simulink model "A5_3_sampling_100ms"  (Simulink 7.4)
settings: Solver=FixedStepDiscrete  StartTime=0.0  StopTime=5  RelTol=1e-3
undefined symbols (not defined in the file): den, num
libraries: DCmotor_library x1
settings Model: Creator=Natalia  LastModifiedBy=ma
settings DebuggingCC: FcnCallInpInsideContextMsg=Enable All  StrictBusMsg=ErrorLevel1
settings HardwareCC: ProdIntDivRoundTo=Zero  ProdEndianess=LittleEndian  ProdHWDeviceType=Generic->32-bit x86 compatible
settings RTWCC: SystemTargetFile=rtwin.tlc  TemplateMakefile=rtwin.tmf  Description=Real-Time Windows Target  ProcessScript=rtwin_make_rtw_hook  RTWCompilerOptimization=On
settings CodeAppCC: MaxIdLength=95  CustomSymbolStrType=$N$R$M_T
settings TargetCC: TargetLibSuffix=_rtwin.lib  TargetPreCompLibLocation=C:\Program Files\MATLAB\R2012a\toolbox\rtw\targets\rtwin\lib\win64  TargetFunctionLibrary=ANSI_C  IsPILTarget=off  MatFileLogging=on  EnableShiftOperators=on
settings CustomProperty: DataType=string  Value=C:/PROGRA~1/MATLAB/R2012a/toolbox/rtw/targets/rtwin

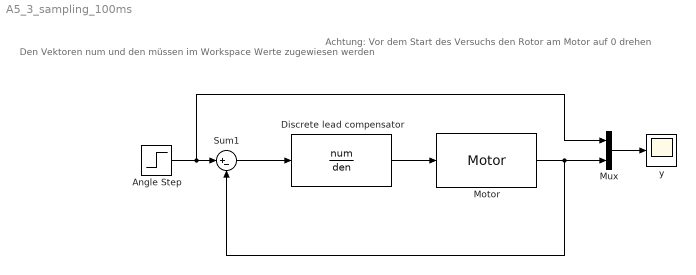
== system A5_3_sampling_100ms ==
  note: Den Vektoren
      | num und den
      | müssen im Workspace
      | Werte zugewiesen werden
  note: Achtung:
      | Vor dem Start des Versuchs
      | den Rotor am Motor auf 0 drehen
  Angle Step : Step  After=2*pi  SampleTime=0.1
  Discrete lead compensator : DiscreteTransferFcn  Numerator=num  Denominator=den  SampleTime=0.1
  Motor : DCmotor_library/Motor  motoridinput=8  name_signal=Angle  ts=100
  Mux : Mux  Inputs=2
  Sum1 : Sum  Inputs=|+-
  y : Scope
      settings: YMin=-0.5  YMax=11
  wires:
  Angle Step/1 -> Mux/1, Sum1/1
  Sum1/1 -> Discrete lead compensator/1
  Discrete lead compensator/1 -> Motor/1
  Motor/1 -> Mux/2, Sum1/2
  Mux/1 -> y/1
